simulink model "APF_SoftLanding_Quadrotor"  (R2023a)
settings: Solver=VariableStepAuto  StartTime=0.0  StopTime=120  RelTol=1e-3
values from neighbouring files (symbols this model uses):
  alpha_t = pi/2    (= 1.57079632679)    [Parameters.m]
  d0 = 7    [Parameters.m]
  k1 = 0.1395    [Parameters.m]
  k2 = 0.1784    [Parameters.m]
  k3 = 0.0442    [Parameters.m]
  ka = 0.2    [Parameters.m]
  katt = 10    [Parameters.m]
  kb = 0.6    [Parameters.m]
  kc = 0.4    [Parameters.m]
  krep = 90000    [Parameters.m]
  m = 5    [Parameters.m]
  maxRange = 10    [Parameters.m]
  n = 3    [Parameters.m]
  P_psi_lead = 2    [Parameters.m]
  P_vel_lead = 5    [Parameters.m]
  posHpad = [-25 -25 0]    [Parameters.m]
  Rmin = 0.1    [Parameters.m]
  target = [-25 -25 -5]    [Parameters.m]
  theta_des = pi/4    (= 0.785398163397)    [Parameters.m]
  thresholdLanding = 15    [Parameters.m]
  v_max = 2    [Parameters.m]
  zeta_des = 0    [Parameters.m]
  zGround = -0.15    [Parameters.m]
undefined symbols (not defined in the file or in its folder): Lidar, numobs, obs, platformUAV
libraries: uavsimlib x5, sharedtransform x2, uavalgslib x1, uavutilslib x1
(part 3 of 3)

== matlab function APF_SoftLanding_Quadrotor/Subsystem/MATLAB Function1 ==
function [V_cmd, yaw_cmd, Stop] = APF_Planner_3D( ...
    pos, goal, obs, katt, krep, safeDist, v_max, numObs)

% =========================================================
% 3D Artificial Potential Field (APF) Planner
% =========================================================
%
% Coordinate system:
%       NED = [North East Down]
%
% INPUT:
%   pos      : UAV position [N E D]
%   goal     : Goal position [N E D]
%   obs      : Obstacle centers, Nx3 [N E D]
%   katt     : Attractive gain
%   krep     : Repulsive gain
%   safeDist : Safety/influence distance from obstacle surface [m]
%   v_max    : Maximum UAV velocity [m/s]
%   numObs   : Number of obstacles
%
% OUTPUT:
%   V_cmd    : Desired velocity [VN VE VD] [m/s]
%   yaw_cmd  : Desired yaw [rad]
%   Stop     : 1 = goal reached
%
% =========================================================

%% --------------------------------------------------------
% 1. Parameters
% ---------------------------------------------------------

% Radius of each spherical obstacle
R_obs = 5.0;       % [m]

% Tangential force gain
k_tan = 0.3*krep;

% Minimum numerical distance
d_min = 0.05;      % [m]

% Goal tolerance
goal_tol = 0.15;   % [m]

% Velocity tolerance near goal
v_min = 0.05;      % [m/s]


%% --------------------------------------------------------
% 2. Initialize fixed-size outputs
% ---------------------------------------------------------

V_cmd   = zeros(1,3);
yaw_cmd = 0.0;
Stop    = 0.0;

F_att   = zeros(1,3);
F_rep   = zeros(1,3);
F_tan   = zeros(1,3);
F_total = zeros(1,3);


%% --------------------------------------------------------
% 3. Convert inputs to fixed-size vectors
% ---------------------------------------------------------

p = zeros(1,3);
g = zeros(1,3);

p(1) = pos(1);
p(2) = pos(2);
p(3) = pos(3);

g(1) = goal(1);
g(2) = goal(2);
g(3) = goal(3);

v_lim = v_max(1);


%% --------------------------------------------------------
% 4. Distance to goal
% ---------------------------------------------------------

d_goal_vec = g - p;

d_goal = sqrt( ...
    d_goal_vec(1)^2 + ...
    d_goal_vec(2)^2 + ...
    d_goal_vec(3)^2 );


%% --------------------------------------------------------
% 5. Goal reached
% ---------------------------------------------------------

if d_goal < goal_tol

    V_cmd(1) = 0.0;
    V_cmd(2) = 0.0;
    V_cmd(3) = 0.0;

    yaw_cmd = 0.0;
    Stop = 1.0;

else

    %% ----------------------------------------------------
    % 6. Attractive force
    % -----------------------------------------------------

    F_att(1) = 2*katt*d_goal_vec(1);
    F_att(2) = 2*katt*d_goal_vec(2);
    F_att(3) = 2*katt*d_goal_vec(3);


    %% ----------------------------------------------------
    % 7. Repulsive force from multiple obstacles
    % -----------------------------------------------------

    for i = 1:numObs

        % -----------------------------------------------
        % Obstacle center
        % -----------------------------------------------

        obs_i = zeros(1,3);

        obs_i(1) = obs(i,1);
        obs_i(2) = obs(i,2);
        obs_i(3) = obs(i,3);


        % -----------------------------------------------
        % Vector from obstacle center to UAV
        % -----------------------------------------------

        d_vec = p - obs_i;

        d_center = sqrt( ...
            d_vec(1)^2 + ...
            d_vec(2)^2 + ...
            d_vec(3)^2 );


        % -----------------------------------------------
        % Avoid division by zero
        % -----------------------------------------------

        if d_center < d_min
            d_center = d_min;
        end


        % -----------------------------------------------
        % Unit vector pointing away from obstacle
        % -----------------------------------------------

        grad_d = zeros(1,3);

        grad_d(1) = d_vec(1)/d_center;
        grad_d(2) = d_vec(2)/d_center;
        grad_d(3) = d_vec(3)/d_center;


        % -----------------------------------------------
        % Distance from UAV to obstacle SURFACE
        %
        % d_surface > 0 : UAV outside obstacle
        % d_surface = 0 : UAV on obstacle surface
        % d_surface < 0 : UAV inside obstacle
        % -----------------------------------------------

        d_surface = d_center - R_obs;


        % -----------------------------------------------
        % Repulsive force
        % Only active inside influence region
        % -----------------------------------------------

        if d_surface < safeDist

            % Prevent singularity
            d_eff = max(d_surface, d_min);


            % -------------------------------------------
            % Repulsive magnitude
            % -------------------------------------------

            rep_mag = 2*krep * ...
                (1/d_eff - 1/safeDist) * ...
                (1/(d_eff^2));


            % -------------------------------------------
            % Repulsive force
            % -------------------------------------------

            F_rep(1) = F_rep(1) + ...
                rep_mag*grad_d(1);

            F_rep(2) = F_rep(2) + ...
                rep_mag*grad_d(2);

            F_rep(3) = F_rep(3) + ...
                rep_mag*grad_d(3);


            % -------------------------------------------
            % 3D Tangential force
            %
            % Project goal direction onto the plane
            % perpendicular to obstacle radial direction.
            % -------------------------------------------

            if d_goal > d_min

                goal_dir = zeros(1,3);

                goal_dir(1) = d_goal_vec(1)/d_goal;
                goal_dir(2) = d_goal_vec(2)/d_goal;
                goal_dir(3) = d_goal_vec(3)/d_goal;


                % Projection of goal direction onto
                % tangent plane of obstacle
                dot_val = ...
                    goal_dir(1)*grad_d(1) + ...
                    goal_dir(2)*grad_d(2) + ...
                    goal_dir(3)*grad_d(3);


                tan_dir = zeros(1,3);

                tan_dir(1) = goal_dir(1) ...
                    - dot_val*grad_d(1);

                tan_dir(2) = goal_dir(2) ...
                    - dot_val*grad_d(2);

                tan_dir(3) = goal_dir(3) ...
                    - dot_val*grad_d(3);


                tan_norm = sqrt( ...
                    tan_dir(1)^2 + ...
                    tan_dir(2)^2 + ...
                    tan_dir(3)^2 );


                % ---------------------------------------
                % If goal direction is almost radial,
                % choose another 3D tangent direction.
                % ---------------------------------------

                if tan_norm > 1e-3

                    tan_dir(1) = tan_dir(1)/tan_norm;
                    tan_dir(2) = tan_dir(2)/tan_norm;
                    tan_dir(3) = tan_dir(3)/tan_norm;

                else

                    % Choose reference axis that is least
                    % parallel to grad_d

                    if abs(grad_d(3)) < 0.9

                        ref = [0,0,1];

                    else

                        ref = [0,1,0];

                    end


                    % Cross product gives a true 3D
                    % tangent direction

                    tan_dir(1) = ...
                        ref(2)*grad_d(3) ...
                        - ref(3)*grad_d(2);

                    tan_dir(2) = ...
                        ref(3)*grad_d(1) ...
                        - ref(1)*grad_d(3);

                    tan_dir(3) = ...
                        ref(1)*grad_d(2) ...
                        - ref(2)*grad_d(1);


                    tan_norm = sqrt( ...
                        tan_dir(1)^2 + ...
                        tan_dir(2)^2 + ...
                        tan_dir(3)^2 );


                    if tan_norm > 1e-3

                        tan_dir(1) = tan_dir(1)/tan_norm;
                        tan_dir(2) = tan_dir(2)/tan_norm;
                        tan_dir(3) = tan_dir(3)/tan_norm;

                    else

                        tan_dir = [0,1,0];

                    end

                end


                % ---------------------------------------
                % Tangential force decreases near
                % obstacle boundary
                % ---------------------------------------

                tan_mag = k_tan * ...
                    (1/d_eff - 1/safeDist);


                F_tan(1) = F_tan(1) + ...
                    tan_mag*tan_dir(1);

                F_tan(2) = F_tan(2) + ...
                    tan_mag*tan_dir(2);

                F_tan(3) = F_tan(3) + ...
                    tan_mag*tan_dir(3);

            end

        end

    end


    %% ----------------------------------------------------
    % 8. Total APF force
    % -----------------------------------------------------

    F_total(1) = ...
        F_att(1) + F_rep(1) + F_tan(1);

    F_total(2) = ...
        F_att(2) + F_rep(2) + F_tan(2);

    F_total(3) = ...
        F_att(3) + F_rep(3) + F_tan(3);


    %% ----------------------------------------------------
    % 9. Convert APF force to velocity command
    %
    % V = Kv * F
    %
    % then saturate to Vmax
    % -----------------------------------------------------

    F_norm = sqrt( ...
        F_total(1)^2 + ...
        F_total(2)^2 + ...
        F_total(3)^2 );


    if F_norm > 1e-4

        % Proportional conversion from force to velocity
        K_v = 1.0;

        V_mag = K_v * F_norm;


        % Saturate velocity
        if V_mag > v_lim

            V_mag = v_lim;

        end


        % Velocity direction
        V_cmd(1) = ...
            V_mag * F_total(1)/F_norm;

        V_cmd(2) = ...
            V_mag * F_total(2)/F_norm;

        V_cmd(3) = ...
            V_mag * F_total(3)/F_norm;

    else

        V_cmd(1) = 0.0;
        V_cmd(2) = 0.0;
        V_cmd(3) = 0.0;

    end


    %% ----------------------------------------------------
    % 10. Slow down near goal
    % -----------------------------------------------------

    if d_goal < 2.0

        scale = d_goal / 2.0;

        if scale < 0.1
            scale = 0.1;
        end

        V_cmd(1) = scale*V_cmd(1);
        V_cmd(2) = scale*V_cmd(2);
        V_cmd(3) = scale*V_cmd(3);

    end


    %% ----------------------------------------------------
    % 11. Yaw command
    %
    % UAV points in direction of horizontal velocity
    % -----------------------------------------------------

    V_horizontal = sqrt( ...
        V_cmd(1)^2 + ...
        V_cmd(2)^2 );


    if V_horizontal > v_min

        yaw_cmd = atan2( ...
            V_cmd(2), ...
            V_cmd(1) );

    else

        yaw_cmd = atan2( ...
            d_goal_vec(2), ...
            d_goal_vec(1) );

    end

end

end

== matlab function APF_SoftLanding_Quadrotor/GuidanceLaw ==
function [dVp_cmd, dalpha_p_cmd, dgamma_cmd, validGuidance] = GuidanceLaw( ...
    Vp, Vt, dVt, alpha_p, gamma, ...
    alpha_t, dalpha_t, ddalpha_t, ...
    Rxy, dRxy, psi, dpsi, S, theta_des, ...
    ka, kb, kc, k1, k2, k3, n, m, validLOS)

% Phase-2 landing guidance. S must use the relative-azimuth surface.
% Angles: rad; rates: rad/s; speeds: m/s; distances: m.
% gamma is positive upward. psi is the LOS azimuth.
% validLOS is the scalar logical output from LOSRate.
% validGuidance reports numerical success, including saturated commands.

% Initialize outputs before every possible early return.
dVp_cmd = 0;
dalpha_p_cmd = 0;
dgamma_cmd = 0;
validGuidance = false;

% Reject the numerical fallback from LOSRate before building A or B.
if ~validLOS
    return;
end

if ~isfinite(Rxy) || Rxy <= 0
    return;
end

if ~isfinite(Vp) || ~isfinite(gamma)
    return;
end

cg = cos(gamma);
sg = sin(gamma);
if Vp <= 1e-6 || abs(cg) <= 1e-6
    return;
end

% The paper uses odd positive n,m with 0 < n < m.
if ~isfinite(n) || ~isfinite(m) || n <= 0 || m <= n
    return;
end
power = n / m;
Sp = sign(S) .* abs(S).^power;

dp = alpha_p - psi;
dt = alpha_t - psi;
td = tan(theta_des);

% Equations (21)-(22).
Ap = [-cos(dp)*cg, Vp*sin(dp)*cg, Vp*cos(dp)*sg; ...
      -sg,          0,             -Vp*cg; ...
      -sin(dp)*cg, -Vp*cos(dp)*cg,  Vp*sin(dp)*sg];
M = [1, 0, 0; td, 1, 0; 0, 0, 1];
A = M * Ap;

% Equation (23), using signed powers of the sliding variables.
dRxy_model = Vt*cos(dt) - Vp*cg*cos(dp);
Fxy = Vp*sin(dp)*cg*dpsi ...
    - dVt*cos(dt) ...
    + Vt*sin(dt)*(dalpha_t - dpsi);

B1 = -k1*Sp(1) + Fxy - ka*dRxy_model;
B2 = td*(Fxy - kb*dRxy_model) - k2*Sp(2) + kb*Vp*sg;
B3 = -Rxy*k3*Sp(3) - kc*Rxy*(dpsi - dalpha_t) ...
    + ddalpha_t*Rxy + dRxy*dpsi ...
    - Vp*cos(dp)*cg*dpsi ...
    - Vt*cos(dt)*(dalpha_t - dpsi) - dVt*sin(dt);
B = [B1; B2; B3];

if ~all(isfinite(A(:))) || ~all(isfinite(B(:)))
    return;
end
if rcond(A) <= 1e-12
    return;
end

Uraw = A \ B;
if ~all(isfinite(Uraw))
    return;
end
dVp = Uraw(1);
dalpha_p = Uraw(2);
dgamma = Uraw(3);

% Algorithm 1 thresholds and symmetric command limits.
M1 = 0.1;
M2 = 0.15;
N1 = 10;
N2 = pi/2;
N3 = pi/2;

if Vp < M1 && dVp < 0
    dVp = 0;
end
if cg < M2 && gamma*dgamma > 0
    dgamma = 0;
end

dVp_cmd = min(N1, max(-N1, dVp));
dalpha_p_cmd = min(N2, max(-N2, dalpha_p));
dgamma_cmd = min(N3, max(-N3, dgamma));
validGuidance = true;
end


%% ========================================================================

% function [dVp_cmd, dalpha_p_cmd, dgamma_cmd] = GuidanceLaw( ...
%     Vp, Vt, dVt, alpha_p, gamma, ...
%     alpha_t, dalpha_t, ddalpha_t, ...
%     Rxy, dRxy, psi, dpsi, S, theta_des, ...
%     ka, kb, kc, k1, k2, k3, n, m)
% 
% % S: 3-by-1 vector [S1; S2; S3], from equation (17).
% % All angles: rad.
% % Angular rates: rad/s.
% % ddalpha_t: rad/s^2.
% % Speeds: m/s. Accelerations: m/s^2.
% %
% % gamma follows the paper convention: positive upward.
% % psi is the LOS azimuth, NOT the UAV body yaw.
% 
% %% Sliding surface
% 
% 
% % Real-valued signed powers.
% % n and m must be odd positive integers, with 0 < n < m.
% power = n / m;
% 
% 
% %% Equation (22): Ap
% Ap = [-cos(alpha_p - psi) * cos(gamma), Vp * sin(alpha_p - psi) * cos(gamma), Vp * cos(alpha_p - psi)*sin(gamma);
%     -sin(gamma), 0, -Vp*cos(gamma);
%     -sin(alpha_p - psi) * cos(gamma), -Vp * cos(alpha_p - psi) * cos(gamma), Vp * sin(alpha_p - psi) * sin(gamma)];
% 
% %% Equation (21): A
% M = [1,  0,  0;
%     tan(theta_des), 1,  0;
%     0,  0,  1];
% 
% A = M * Ap;
% 
% %% Equation (23): B
% 
% B1 = -k1 * abs(S(1))^power + Vp * sin(alpha_p - psi) * cos(gamma) * dpsi...
%     -dVt * cos(alpha_t -psi) + Vt * sin(alpha_t - psi) * (dalpha_t - dpsi)...
%     - ka * (Vt * cos(alpha_t - psi) - Vp * cos(gamma) * cos(alpha_p - psi));
% 
% B2 = tan(theta_des) * (Vp * sin(alpha_p - psi) * cos(gamma) * dpsi...
%      - dVt * cos(alpha_t - psi) + Vt  * sin(alpha_t - psi) * (dalpha_t - dpsi)...
%      - kb * (Vt * cos(alpha_t - psi) - Vp * cos(gamma) * cos(alpha_p - psi)))...
%      - k2 * abs(S(2))^power + kb * Vp*sin(gamma);
% 
% B3 = -Rxy * k3 * abs(S(3))^power - kc * Rxy * (dpsi - dalpha_t) ...
%      + ddalpha_t * Rxy + dRxy * dpsi - Vp * cos(alpha_p - psi) * cos(gamma) * dpsi ...
%      - Vt * cos(alpha_t - psi)*(dalpha_t - dpsi) - dVt * sin(alpha_t - psi);
% 
% B = [B1; B2; B3];
% 
% %% Algorithm 1 parameters
% % Values used in the paper's point-mass simulations
% M1 = 0.1;       % Speed threshold, m/s
% M2 = 0.15;      % Threshold for cos(gamma), dimensionless
% 
% N1 = 10;        % Maximum |dVp|, m/s^2
% N2 = pi/2;      % Maximum |dalpha_p|, rad/s
% N3 = pi/2;      % Maximum |dgamma|, rad/s
% 
% %% Additional numerical protection BEFORE solving A*U = B
% % These checks are implementation additions, not Algorithm 1.
% valid = false;
% 
% dVp_cmd      = 0;
% dalpha_p_cmd = 0;
% dgamma_cmd   = 0;
% 
% if ~all(isfinite(A(:))) || ~all(isfinite(B(:)))
%     return;
% end
% 
% if Vp <= 1e-6 || abs(cos(gamma)) <= 1e-6
%     return;
% end
% 
% if rcond(A) <= 1e-12
%     return;
% end
% 
% %% Equation (24)
% Uraw = A \ B;
% 
% if ~all(isfinite(Uraw))
%     return;
% end
% 
% dVp      = Uraw(1);
% dalpha_p = Uraw(2);
% dgamma   = Uraw(3);
% 
% %% Algorithm 1: prevent further speed reduction
% if Vp < M1 && dVp < 0
%     dVp = 0;
% end
% 
% %% Algorithm 1: prevent motion toward vertical flight
% % The paper uses: cos(gamma) < M2 && gamma*dgamma > 0
% if cos(gamma) < M2 && gamma*dgamma > 0
%     dgamma = 0;
% end
% 
% %% Symmetric command limits
% dVp_cmd      = min(N1, max(-N1, dVp));
% dalpha_p_cmd = min(N2, max(-N2, dalpha_p));
% dgamma_cmd   = min(N3, max(-N3, dgamma));
% 
% valid = true;
% 
% %% Equation (24): U = inv(A)*B
% % Solve the linear system instead of explicitly computing inv(A).
% % U = A \ B;
% % 
% % dVp_cmd      = U(1);
% % dalpha_p_cmd = U(2);
% % dgamma_cmd   = U(3);
% 
% end
